simulink model "Target_Control_System"  (R2021b)
settings: Solver=FixedStepDiscrete  StartTime=0.0  StopTime=5  RelTol=1e-3
PreLoadFcn:
  | RTWConfigurationCB('preloadfcn', bdroot);
PostLoadFcn:
  | load('configuration/data_struct.mat');
  | load('configuration/fluxMaps_propMotor.mat');
  | load('configuration/parameterInit_PROP.mat');
  | load('configuration/parameterInit_PUMP.mat');
  | load('configuration/parameterInit_PITCH.mat');
  | load('configuration/parameterInit_TILT.mat');
  | %load('configuration/base_workspace_signal_definition.mat');
  | %load('resolvedatastores_to_baseworkspace_for_faster_simulation.mat');
model workspace (MAT data in the model file):
  SIMULATION_OPTIONS : Simulink.Parameter (value not decoded)
  TARGET_CODE_GEN : Simulink.Parameter (value not decoded)
  TCS_SAMPLE_FREQ_HZ : Simulink.Parameter (value not decoded)
symbols that are objects in the model workspace (value not decoded): TARGET_CODE_GEN, TCS_SAMPLE_FREQ_HZ
undefined symbols (not defined in the file): A_DQ_REF_LPF_INIT__PITCH, A_DQ_REF_LPF_INIT__PROP, A_DQ_REF_LPF_INIT__PUMP, A_DQ_REF_LPF_INIT__TILT, A_OBSERVER_CONFIDENCE_INIT__PITCH, A_OBSERVER_CONFIDENCE_INIT__PROP, A_OBSERVER_CONFIDENCE_INIT__PUMP, A_OBSERVER_CONFIDENCE_INIT__TILT, ACTUATOR_MAX_ANGLE_TRIP__PITCH, ACTUATOR_MIN_ANGLE_TRIP__PITCH, ACTUATOR_POS_SENSOR_INV_DIRECTION__PITCH, ACTUATOR_POS_SENSOR_INV_DIRECTION__TILT, ACTUATOR_POS_SENSOR_OFFSET__PITCH, ACTUATOR_POS_SENSOR_OFFSET__TILT, ADC_scaler1_baseaddr_TILT, ADC_SCALER_FLOAT_TO_FIXPOINT_EXPANSION, ANGLE_ELEC_FROM_SENSOR_OFFSET_INIT__PITCH, ANGLE_ELEC_FROM_SENSOR_OFFSET_INIT__PROP, ANGLE_ELEC_FROM_SENSOR_OFFSET_INIT__PUMP, ANGLE_ELEC_FROM_SENSOR_OFFSET_INIT__TILT, AUTO_CLEAR_FAULTS_ENABLED__PITCH, AUTO_CLEAR_FAULTS_ENABLED__PROP, AUTO_CLEAR_FAULTS_ENABLED__PUMP, AUTO_CLEAR_FAULTS_ENABLED__TILT, AUTO_CLEAR_FAULTS_WAIT_TICKS__PITCH, AUTO_CLEAR_FAULTS_WAIT_TICKS__PROP, AUTO_CLEAR_FAULTS_WAIT_TICKS__PUMP, AUTO_CLEAR_FAULTS_WAIT_TICKS__TILT, AUTO_I_ZERO_IDLE_TICKS__PITCH, AUTO_I_ZERO_IDLE_TICKS__PROP, AUTO_I_ZERO_IDLE_TICKS__PUMP, AUTO_I_ZERO_IDLE_TICKS__TILT, AUTO_I_ZERO_OFFSET_IDC_THRESHOLD__PITCH, AUTO_I_ZERO_OFFSET_IDC_THRESHOLD__PROP, AUTO_I_ZERO_OFFSET_IDC_THRESHOLD__PUMP, AUTO_I_ZERO_OFFSET_IDC_THRESHOLD__TILT, AUTO_I_ZERO_OFFSET_IPH_THRESHOLD__PITCH, AUTO_I_ZERO_OFFSET_IPH_THRESHOLD__PROP, AUTO_I_ZERO_OFFSET_IPH_THRESHOLD__PUMP, AUTO_I_ZERO_OFFSET_IPH_THRESHOLD__TILT, AUTO_SENSORLESS_SWITCHOVER_DISABLE_OMEGA, AUTO_SENSORLESS_SWITCHOVER_ENABLE_OMEGA, AUTO_SENSORLESS_SWITCHOVER_MIN_CONFIDENCE, AUXILIARY_PROTECTION_UNIT_BASEADDR__TILT, blanking_max_error_omega_INIT_PITCH, blanking_max_error_omega_INIT_TILT, blanking_max_error_position_INIT_PITCH, blanking_max_error_position_INIT_TILT, BRUTE_START_I_Q_REF_RAMP_SPEED__PITCH, BRUTE_START_I_Q_REF_RAMP_SPEED__PROP, BRUTE_START_I_Q_REF_RAMP_SPEED__PUMP, BRUTE_START_I_Q_REF_RAMP_SPEED__TILT, CONTROL_LOOP_DT_INIT__PITCH, CONTROL_LOOP_DT_INIT__PROP, CONTROL_LOOP_DT_INIT__PUMP, CONTROL_LOOP_DT_INIT__TILT, CORRECTION_FILTER_SCALE__PITCH, CORRECTION_FILTER_SCALE__PROP, CORRECTION_FILTER_SCALE__PUMP, CORRECTION_FILTER_SCALE__TILT ... (+458)
libraries: simulink x178, Reusables_Lib x24
(part 8 of 47)

== system Target_Control_System/Target_Control_System/InterruptFunction/tiltMotor_isrSchedule/Triggered Subsystem ==
  Trigger : TriggerPort  VariantControl=Variant
  Data Store Write6 : DataStoreWrite  Commented=on  DataStoreName=mdl_suiIsrSmallInvCounter_  IndexOptions=Index vector (dialog)  Indices=1  OutputSizes=1
  Function-Call Generator : simulink/Ports & Subsystems/Function-Call Generator  sample_time=-1  numberOfIterations=1  DisallowWideOutput=off
  constant : Constant  Commented=on  OutDataTypeStr=uint32  SampleTime=-1
  Output : Outport
  wires:
  constant/1 -> Data Store Write6/1
  Function-Call Generator/1 -> Output/1

== system Target_Control_System/Target_Control_System/InterruptFunction/tiltMotor_isrTask/abcToAlphaBeta ==
  abcToAlphaBeta : TriggerPort  TriggerType=function-call  VariantControl=Variant
  Alpha-Beta Calcs : Subsystem
  Calc Angle From Speed : Subsystem
  Constant1 : Constant  Value=TARGET_CODE_GEN  SampleTime=-1
  Data Store Read1 : DataStoreRead  DataStoreName=oTilt  DataStoreElements=oTilt.oIsr_.oIn_.oAdcData_.fIa_  IndexOptions=Index vector (dialog)  Indices=1  OutputSizes=1
  Data Store Read13 : DataStoreRead  DataStoreName=oTilt  DataStoreElements=oTilt.oIsr_.oParam_.iInverseDirection_  IndexOptions=Index vector (dialog)  Indices=1  OutputSizes=1
  Data Store Read14 : DataStoreRead  DataStoreName=oTilt  DataStoreElements=oTilt.oIsr_.oState_.fUaPostlpf_  IndexOptions=Index vector (dialog)  Indices=1  OutputSizes=1
  Data Store Read15 : DataStoreRead  DataStoreName=oTilt  DataStoreElements=oTilt.oIsr_.oState_.fUbPostlpf_  IndexOptions=Index vector (dialog)  Indices=1  OutputSizes=1
  Data Store Read16 : DataStoreRead  DataStoreName=oTilt  DataStoreElements=oTilt.oIsr_.oState_.fUcPostlpf_  IndexOptions=Index vector (dialog)  Indices=1  OutputSizes=1
  Data Store Read17 : DataStoreRead  DataStoreName=oTilt  DataStoreElements=oTilt.oIsr_.oState_.fOmegaEObserverRaw2_  IndexOptions=Index vector (dialog)  Indices=1  OutputSizes=1
  Data Store Read2 : DataStoreRead  DataStoreName=oTilt  DataStoreElements=oTilt.oIsr_.oIn_.oAdcData_.fIb_  IndexOptions=Index vector (dialog)  Indices=1  OutputSizes=1
  Data Store Read4 : DataStoreRead  DataStoreName=oTilt  DataStoreElements=oTilt.oIsr_.oIn_.oAdcData_.fIc_  IndexOptions=Index vector (dialog)  Indices=1  OutputSizes=1
  Data Store Read8 : DataStoreRead  DataStoreName=oTilt  DataStoreElements=oTilt.oIsr_.oIn_.fUphFilterDelayAngleRad_  IndexOptions=Index vector (dialog)  Indices=1  OutputSizes=1
  Data Store Write1 : DataStoreWrite  DataStoreName=oTilt  DataStoreElements=oTilt.oIsr_.oState_.fFluxMainAngleUltraRaw_  IndexOptions=Index vector (dialog)  Indices=1  OutputSizes=1
  Data Store Write2 : DataStoreWrite  DataStoreName=oTilt  DataStoreElements=oTilt.oIsr_.oState_.fIAlpha_  IndexOptions=Index vector (dialog)  Indices=1  OutputSizes=1
  Data Store Write3 : DataStoreWrite  DataStoreName=oTilt  DataStoreElements=oTilt.oIsr_.oState_.fIBeta_  IndexOptions=Index vector (dialog)  Indices=1  OutputSizes=1
  Data Store Write4 : DataStoreWrite  DataStoreName=oTilt  DataStoreElements=oTilt.oIsr_.oState_.fUAlpha_  IndexOptions=Index vector (dialog)  Indices=1  OutputSizes=1
  Data Store Write6 : DataStoreWrite  DataStoreName=oTilt  DataStoreElements=oTilt.oIsr_.oState_.fUBeta_  IndexOptions=Index vector (dialog)  Indices=1  OutputSizes=1
  ModelSource : Subsystem  Commented=on  Variant=on
  NOT1 : Logic  Operator=NOT  AllPortsSameDT=off  OutDataTypeStr=boolean
  vsincos()1 : Subsystem  TreatAsAtomicUnit=on
  wires:
  Alpha-Beta Calcs/4(fUBeta) -> Data Store Write6/1
  Data Store Read13/1 -> Alpha-Beta Calcs/1(iInverseDirection)
  Data Store Read16/1 -> Alpha-Beta Calcs/7(fUcPostlpf)
  Data Store Read1/1 -> Alpha-Beta Calcs/2(fIa)
  Alpha-Beta Calcs/3(fUAlpha) -> Data Store Write4/1
  Alpha-Beta Calcs/2(fIBeta) -> Data Store Write3/1
  Data Store Read15/1 -> Alpha-Beta Calcs/6(fUbPostlpf)
  Data Store Read17/1 -> Calc Angle From Speed/1(Omega)
  Data Store Read2/1 -> Alpha-Beta Calcs/3(fIb)
  Constant1/1 -> NOT1/1
  Data Store Read4/1 -> Alpha-Beta Calcs/4(fIc)
  Data Store Read8/1 -> vsincos()1/1(fUphFilterDelayAngleRad)
  Calc Angle From Speed/1(fFluxMainAngleRaw2) -> vsincos()1/2(fFluxMainAngleRaw2), Data Store Write1/1
  NOT1/1 -> vsincos()1/Enable
  Data Store Read14/1 -> Alpha-Beta Calcs/5(fUaPostlpf)
  Alpha-Beta Calcs/1(fIAlpha) -> Data Store Write2/1

== system Target_Control_System/Target_Control_System/InterruptFunction/tiltMotor_isrTask/currentController ==
  currentController : TriggerPort  TriggerType=function-call  VariantControl=Variant
  Data Store Read1 : DataStoreRead  DataStoreName=oTilt  DataStoreElements=oTilt.oIsr_.oIn_.uiCurrentControllerActive_  IndexOptions=Index vector (dialog)  Indices=1  OutputSizes=1
  Enabled Subsystem : Subsystem  TreatAsAtomicUnit=on
  wires:
  Data Store Read1/1 -> Enabled Subsystem/Enable

== system Target_Control_System/Target_Control_System/InterruptFunction/tiltMotor_isrTask/dqTransform ==
  dqTransform : TriggerPort  TriggerType=function-call  VariantControl=Variant
  DQ Transform : Subsystem
  Data Store Read4 : DataStoreRead  DataStoreName=oTilt  DataStoreElements=oTilt.oMot_.oParam_.fPolePairs_  IndexOptions=Index vector (dialog)  Indices=1  OutputSizes=1
  Data Store Read5 : DataStoreRead  DataStoreName=oTilt  DataStoreElements=oTilt.oIsr_.oState_.fFluxMainMagnitudeLpf_  IndexOptions=Index vector (dialog)  Indices=1  OutputSizes=1
  Data Store Read6 : DataStoreRead  DataStoreName=oTilt  DataStoreElements=oTilt.oIsr_.oState_.fIq_  IndexOptions=Index vector (dialog)  Indices=1  OutputSizes=1
  Data Store Read8 : DataStoreRead  DataStoreName=oTilt  DataStoreElements=oTilt.oIsr_.oState_.fIAlpha_  IndexOptions=Index vector (dialog)  Indices=1  OutputSizes=1
  Data Store Read9 : DataStoreRead  DataStoreName=oTilt  DataStoreElements=oTilt.oIsr_.oState_.fIBeta_  IndexOptions=Index vector (dialog)  Indices=1  OutputSizes=1
  Data Store Write1 : DataStoreWrite  DataStoreName=oTilt  DataStoreElements=oTilt.oIsr_.oOut_.fTEstimate_  IndexOptions=Index vector (dialog)  Indices=1  OutputSizes=1
  Data Store Write2 : DataStoreWrite  DataStoreName=oTilt  DataStoreElements=oTilt.oIsr_.oState_.fId_  IndexOptions=Index vector (dialog)  Indices=1  OutputSizes=1
  Data Store Write4 : DataStoreWrite  DataStoreName=oTilt  DataStoreElements=oTilt.oIsr_.oState_.fIq_  IndexOptions=Index vector (dialog)  Indices=1  OutputSizes=1
  Data Store Write5 : DataStoreWrite  DataStoreName=oTilt  DataStoreElements=oTilt.oIsr_.oOut_.fIPhaseMagnitude_  IndexOptions=Index vector (dialog)  Indices=1  OutputSizes=1
  Torque_Estimation_Pitch : Subsystem
  wires:
  DQ Transform/1(fId) -> Data Store Write2/1
  Data Store Read9/1 -> DQ Transform/2(fIBeta)
  DQ Transform/2(fIq) -> Data Store Write4/1
  Data Store Read4/1 -> Torque_Estimation_Pitch/1(fPolePairs)
  Torque_Estimation_Pitch/1(fTEstimate) -> Data Store Write1/1
  DQ Transform/3(fIPhaseMagnitude) -> Data Store Write5/1
  Data Store Read5/1 -> Torque_Estimation_Pitch/2(fFluxMainMagnitudeLpf)
  Data Store Read8/1 -> DQ Transform/1(fIAlpha)
  Data Store Read6/1 -> Torque_Estimation_Pitch/3(fIq)

== system Target_Control_System/Target_Control_System/InterruptFunction/tiltMotor_isrTask/fluxAngleCalculation ==
  fluxAngleCalculation : TriggerPort  TriggerType=function-call  VariantControl=Variant
  Advance Forced Angle : Subsystem
  Back Rotation : Subsystem
  Constant5 : Constant  Value=TARGET_CODE_GEN  SampleTime=-1
  Data Store Read10 : DataStoreRead  DataStoreName=oTilt  DataStoreElements=oTilt.oIsr_.oIn_.uiForcedAngle_  IndexOptions=Index vector (dialog)  Indices=1  OutputSizes=1
  Data Store Read2 : DataStoreRead  DataStoreName=oTilt  DataStoreElements=oTilt.oIsr_.oIn_.fOmegaERefRampOut_  IndexOptions=Index vector (dialog)  Indices=1  OutputSizes=1
  Data Store Read3 : DataStoreRead  DataStoreName=oTilt  DataStoreElements=oTilt.oIsr_.oParam_.iUseSensorAngle_  IndexOptions=Index vector (dialog)  Indices=1  OutputSizes=1
  Data Store Read4 : DataStoreRead  DataStoreName=oTilt  DataStoreElements=oTilt.oIsr_.oIn_.fFluxMasterAngleForced2closedSmoothingRampOut_  IndexOptions=Index vector (dialog)  Indices=1  OutputSizes=1
  Data Store Read5 : DataStoreRead  DataStoreName=oTilt  DataStoreElements=oTilt.oIsr_.oIn_.fOmegaElecFromPosSensor_  IndexOptions=Index vector (dialog)  Indices=1  OutputSizes=1
  Data Store Read6 : DataStoreRead  DataStoreName=oTilt  DataStoreElements=oTilt.oIsr_.oIn_.fFluxMasterAngleOffsetRampOut_  IndexOptions=Index vector (dialog)  Indices=1  OutputSizes=1
  Data Store Read7 : DataStoreRead  DataStoreName=oTilt  DataStoreElements=oTilt.oIsr_.oState_.fOmegaEObserverLpf2_  IndexOptions=Index vector (dialog)  Indices=1  OutputSizes=1
  Data Store Read8 : DataStoreRead  DataStoreName=oTilt  DataStoreElements=oTilt.oIsr_.oIn_.fAngleElecFromPosSensor_  IndexOptions=Index vector (dialog)  Indices=1  OutputSizes=1
  Data Store Read9 : DataStoreRead  DataStoreName=oTilt  DataStoreElements=oTilt.oIsr_.oState_.fFluxMainAngleRaw2_  IndexOptions=Index vector (dialog)  Indices=1  OutputSizes=1
  Data Store Write21 : DataStoreWrite  DataStoreName=mdl_tilt_fOmegaE  IndexOptions=Index vector (dialog)  Indices=1  OutputSizes=1
  Data Store Write3 : DataStoreWrite  DataStoreName=oTilt  DataStoreElements=oTilt.oIsr_.oState_.fFluxMasterAngleBkwd_  IndexOptions=Index vector (dialog)  Indices=1  OutputSizes=1
  Data Store Write4 : DataStoreWrite  DataStoreName=oTilt  DataStoreElements=oTilt.oIsr_.oState_.fFluxMasterAngle_  IndexOptions=Index vector (dialog)  Indices=1  OutputSizes=1
  Equal4 : RelationalOperator  Operator===  OutDataTypeStr=boolean  RndMeth=Simplest
  ModelSource : Subsystem  Variant=on
  NOT2 : Logic  Operator=NOT  AllPortsSameDT=off  OutDataTypeStr=boolean
  Not forced Angle : Subsystem
  One3 : Constant  OutDataTypeStr=uint32  SampleTime=-1
  Switch1 : Switch  Criteria=u2 > Threshold  Threshold=0.5
  Switch2 : Switch  Criteria=u2 > Threshold  Threshold=0.5
  vsincos() : Subsystem  TreatAsAtomicUnit=on
  wires:
  Constant5/1 -> NOT2/1
  Advance Forced Angle/1(Output) -> Switch2/1
  Data Store Read2/1 -> Advance Forced Angle/1(Input), Switch1/1
  Equal4/1 -> Switch1/2, Switch2/2
  Data Store Read3/1 -> Not forced Angle/1(iUseSensorAngle)
  Switch2/1 -> Data Store Write4/1, vsincos()/2(fFluxMasterAngle), Back Rotation/2(fFluxMasterAngle)
  Data Store Read6/1 -> Back Rotation/1(fFluxMasterAngleOffsetRampOut)
  One3/1 -> Equal4/2
  Data Store Read4/1 -> Not forced Angle/6(fFluxMasterAngleForced2closedSmoothingRampOut)
  Data Store Read5/1 -> Not forced Angle/4(fOmegaElecFromPosSensor)
  Data Store Read7/1 -> Not forced Angle/5(fOmegaEObserverLpf2)
  Data Store Read9/1 -> Not forced Angle/3(fFluxMainAngleRaw2)
  Data Store Read8/1 -> Not forced Angle/2(fAngleElecFromPosSensor)
  Data Store Read10/1 -> Equal4/1
  Not forced Angle/1(fFluxMasterAngle) -> Switch2/3
  Back Rotation/1(fFluxMasterAngleBkwd) -> Data Store Write3/1, vsincos()/1(fFluxMasterAngleBkwd)
  Switch1/1 -> Data Store Write21/1
  NOT2/1 -> vsincos()/Enable
  Not forced Angle/2(fOmegaE) -> Switch1/3

== system Target_Control_System/Target_Control_System/InterruptFunction/tiltMotor_isrTask/fluxObserver ==
  fluxObserver : TriggerPort  TriggerType=function-call  VariantControl=Variant
  Calculate Coil Flux + Bleeder : Subsystem
  Calculate Main Flux + LPF : Subsystem
  Data Store Read : DataStoreRead  DataStoreName=oTilt  DataStoreElements=oTilt.oIsr_.oParam_.fRsPhase_  IndexOptions=Index vector (dialog)  Indices=1  OutputSizes=1
  Data Store Read1 : DataStoreRead  DataStoreName=oTilt  DataStoreElements=oTilt.oIsr_.oIn_.fUphFilterAmplitudeRatio_  IndexOptions=Index vector (dialog)  Indices=1  OutputSizes=1
  Data Store Read10 : DataStoreRead  DataStoreName=oTilt  DataStoreElements=oTilt.oIsr_.oParam_.fLsPhase_  IndexOptions=Index vector (dialog)  Indices=1  OutputSizes=1
  Data Store Read11 : DataStoreRead  DataStoreName=oTilt  DataStoreElements=oTilt.oMot_.oParam_.fObserverLoopFilterBandwidthHz_  IndexOptions=Index vector (dialog)  Indices=1  OutputSizes=1
  Data Store Read12 : DataStoreRead  DataStoreName=oTilt  DataStoreElements=oTilt.oIsr_.oParam_.oPiDataPll2_.fState_  IndexOptions=Index vector (dialog)  Indices=1  OutputSizes=1
  Data Store Read13 : DataStoreRead  DataStoreName=oTilt  DataStoreElements=oTilt.oIsr_.oParam_.oPiDataPll2_.oParameter_.fKp_  IndexOptions=Index vector (dialog)  Indices=1  OutputSizes=1
  Data Store Read14 : DataStoreRead  DataStoreName=oTilt  DataStoreElements=oTilt.oIsr_.oParam_.oPiDataPll2_.oParameter_.fKi_  IndexOptions=Index vector (dialog)  Indices=1  OutputSizes=1
  Data Store Read15 : DataStoreRead  DataStoreName=oTilt  DataStoreElements=oTilt.oIsr_.oParam_.oPiDataPll2_.oParameter_.fLoopDt_  IndexOptions=Index vector (dialog)  Indices=1  OutputSizes=1
  Data Store Read16 : DataStoreRead  DataStoreName=oTilt  DataStoreElements=oTilt.oIsr_.oParam_.oPiDataPll2_.oParameter_.fIntMax_  IndexOptions=Index vector (dialog)  Indices=1  OutputSizes=1
  Data Store Read17 : DataStoreRead  DataStoreName=oTilt  DataStoreElements=oTilt.oIsr_.oParam_.oPiDataPll2_.oParameter_.fOutMax_  IndexOptions=Index vector (dialog)  Indices=1  OutputSizes=1
  Data Store Read18 : DataStoreRead  DataStoreName=oTilt  DataStoreElements=oTilt.oIsr_.oParam_.oPiDataPll2_.oParameter_.fIntMin_  IndexOptions=Index vector (dialog)  Indices=1  OutputSizes=1
  Data Store Read19 : DataStoreRead  DataStoreName=oTilt  DataStoreElements=oTilt.oIsr_.oParam_.oPiDataPll2_.oParameter_.fOutMin_  IndexOptions=Index vector (dialog)  Indices=1  OutputSizes=1
  Data Store Read2 : DataStoreRead  DataStoreName=mdl_tilt_fFluxMainAngleRaw2_sin_  IndexOptions=Index vector (dialog)  Indices=1  OutputSizes=1
  Data Store Read27 : DataStoreRead  DataStoreName=mdl_tilt_fUphFilterDelayAngleRad_sin_  IndexOptions=Index vector (dialog)  Indices=1  OutputSizes=1
  Data Store Read28 : DataStoreRead  DataStoreName=mdl_tilt_fUphFilterDelayAngleRad_cos_  IndexOptions=Index vector (dialog)  Indices=1  OutputSizes=1
  Data Store Read3 : DataStoreRead  DataStoreName=oTilt  DataStoreElements=oTilt.oIsr_.oParam_.uiUphFilterCorrectionEnabled_  IndexOptions=Index vector (dialog)  Indices=1  OutputSizes=1
  Data Store Read34 : DataStoreRead  DataStoreName=mdl_tilt_fFluxMainAngleRaw2_cos_  IndexOptions=Index vector (dialog)  Indices=1  OutputSizes=1
  Data Store Read4 : DataStoreRead  DataStoreName=oTilt  DataStoreElements=oTilt.oIsr_.oState_.fUAlpha_  IndexOptions=Index vector (dialog)  Indices=1  OutputSizes=1
  Data Store Read5 : DataStoreRead  DataStoreName=oTilt  DataStoreElements=oTilt.oIsr_.oState_.fUBeta_  IndexOptions=Index vector (dialog)  Indices=1  OutputSizes=1
  Data Store Read6 : DataStoreRead  DataStoreName=oTilt  DataStoreElements=oTilt.oIsr_.oState_.fIAlpha_  IndexOptions=Index vector (dialog)  Indices=1  OutputSizes=1
  Data Store Read7 : DataStoreRead  DataStoreName=oTilt  DataStoreElements=oTilt.oIsr_.oState_.fIBeta_  IndexOptions=Index vector (dialog)  Indices=1  OutputSizes=1
  Data Store Read8 : DataStoreRead  DataStoreName=oTilt  DataStoreElements=oTilt.oIsr_.oParam_.fControlLoopDt_  IndexOptions=Index vector (dialog)  Indices=1  OutputSizes=1
  Data Store Read9 : DataStoreRead  DataStoreName=oTilt  DataStoreElements=oTilt.oIsr_.oParam_.fKFluxBleeder_  IndexOptions=Index vector (dialog)  Indices=1  OutputSizes=1
  Data Store Write1 : DataStoreWrite  DataStoreName=oTilt  DataStoreElements=oTilt.oIsr_.oState_.fFluxCoilAlpha_  IndexOptions=Index vector (dialog)  Indices=1  OutputSizes=1
  Data Store Write10 : DataStoreWrite  DataStoreName=oTilt  DataStoreElements=oTilt.oIsr_.oState_.fAtan2loopfilter2Out_  IndexOptions=Index vector (dialog)  Indices=1  OutputSizes=1
  Data Store Write11 : DataStoreWrite  DataStoreName=oTilt  DataStoreElements=oTilt.oIsr_.oParam_.oPiDataPll2_.fState_  IndexOptions=Index vector (dialog)  Indices=1  OutputSizes=1
  Data Store Write12 : DataStoreWrite  DataStoreName=oTilt  DataStoreElements=oTilt.oIsr_.oState_.fOmegaEObserverRaw2_  IndexOptions=Index vector (dialog)  Indices=1  OutputSizes=1
  Data Store Write13 : DataStoreWrite  DataStoreName=oTilt  DataStoreElements=oTilt.oIsr_.oState_.fOmegaEObserverLpf2_  IndexOptions=Index vector (dialog)  Indices=1  OutputSizes=1
  Data Store Write14 : DataStoreWrite  DataStoreName=oTilt  DataStoreElements=oTilt.oIsr_.oState_.fFluxMainMagnitudeLpf_  IndexOptions=Index vector (dialog)  Indices=1  OutputSizes=1
  Data Store Write15 : DataStoreWrite  DataStoreName=oTilt  DataStoreElements=oTilt.oIsr_.oState_.fFluxMainMagnitude_  IndexOptions=Index vector (dialog)  Indices=1  OutputSizes=1
  Data Store Write2 : DataStoreWrite  DataStoreName=oTilt  DataStoreElements=oTilt.oIsr_.oState_.fUBeta_  IndexOptions=Index vector (dialog)  Indices=1  OutputSizes=1
  Data Store Write28 : DataStoreWrite  DataStoreName=oTilt  DataStoreElements=oTilt.oIsr_.oState_.fIAlphaLpf4hpf_  IndexOptions=Index vector (dialog)  Indices=1  OutputSizes=1
  Data Store Write29 : DataStoreWrite  DataStoreName=oTilt  DataStoreElements=oTilt.oIsr_.oState_.fIBetaLpf4hpf_  IndexOptions=Index vector (dialog)  Indices=1  OutputSizes=1
  Data Store Write3 : DataStoreWrite  DataStoreName=oTilt  DataStoreElements=oTilt.oIsr_.oState_.fUAlphaLpf4hpf_  IndexOptions=Index vector (dialog)  Indices=1  OutputSizes=1
  Data Store Write4 : DataStoreWrite  DataStoreName=oTilt  DataStoreElements=oTilt.oIsr_.oState_.fUBetaLpf4hpf_  IndexOptions=Index vector (dialog)  Indices=1  OutputSizes=1
  Data Store Write5 : DataStoreWrite  DataStoreName=oTilt  DataStoreElements=oTilt.oIsr_.oState_.fUAlpha_  IndexOptions=Index vector (dialog)  Indices=1  OutputSizes=1
  Data Store Write6 : DataStoreWrite  DataStoreName=oTilt  DataStoreElements=oTilt.oIsr_.oState_.fFluxCoilBeta_  IndexOptions=Index vector (dialog)  Indices=1  OutputSizes=1
  Data Store Write7 : DataStoreWrite  DataStoreName=oTilt  DataStoreElements=oTilt.oIsr_.oState_.fFluxMainAlpha_  IndexOptions=Index vector (dialog)  Indices=1  OutputSizes=1
  Data Store Write8 : DataStoreWrite  DataStoreName=oTilt  DataStoreElements=oTilt.oIsr_.oState_.fFluxMainBeta_  IndexOptions=Index vector (dialog)  Indices=1  OutputSizes=1
  Data Store Write9 : DataStoreWrite  DataStoreName=oTilt  DataStoreElements=oTilt.oIsr_.oState_.fFluxMainAngleUltraRaw_  IndexOptions=Index vector (dialog)  Indices=1  OutputSizes=1
  Fast PLL : Subsystem
  HPF Currents : Subsystem
  HPF Voltages : Subsystem
  Mux : Mux  Inputs=7
  Subtract Resistive Voltage Drop : Subsystem
  Ultra Raw Angle : Subsystem
  Voltage Vector Rotation : Subsystem
  wires:
  Data Store Read13/1 -> Mux/1
  Data Store Read5/1 -> Voltage Vector Rotation/6(fUBeta)
  Calculate Main Flux + LPF/2(fFluxMainBeta) -> Fast PLL/4(fFluxMainBeta), Ultra Raw Angle/2(fFluxMainBeta), Data Store Write8/1
  Data Store Read11/1 -> Fast PLL/5(fObserverLoopFilterBandwidthHz)
  Voltage Vector Rotation/2(fUBeta_out) -> Subtract Resistive Voltage Drop/5(fUBeta)
  Data Store Read34/1 -> Fast PLL/2(fluxAngle_cos)
  Data Store Read27/1 -> Voltage Vector Rotation/1(UphFilterDelayAngleRad_sin)
  Fast PLL/1(fAtan2loopfilter2Out) -> Data Store Write10/1
  HPF Currents/2(fIBetaLpf4hpf) -> Data Store Write29/1
  Calculate Coil Flux + Bleeder/1(fFluxCoilAlpha) -> Calculate Main Flux + LPF/4(fFluxCoilAlpha), Data Store Write1/1
  Data Store Read14/1 -> Mux/2
  Data Store Read3/1 -> Voltage Vector Rotation/4(uiUphFilterCorrectionEnabled)
  Data Store Read10/1 -> Calculate Main Flux + LPF/3(fLsPhase)
  Data Store Read7/1 -> HPF Currents/2(fIBeta)
  Data Store Read1/1 -> Voltage Vector Rotation/3(fUphFilterAmplitudeRatio)
  Data Store Read2/1 -> Fast PLL/1(fluxAngle_sin)
  Data Store Read/1 -> Subtract Resistive Voltage Drop/3(fRsPhase)
  HPF Currents/4(fIBetaLocal) -> Calculate Main Flux + LPF/2(fIBetaLocal), Subtract Resistive Voltage Drop/2(fIBetaLocal)  "fIBetaLocal"
  Data Store Read18/1 -> Mux/6
  Calculate Coil Flux + Bleeder/2(fFluxCoilBeta) -> Calculate Main Flux + LPF/5(fFluxCoilBeta), Data Store Write6/1
  Calculate Main Flux + LPF/3(fFluxMainMagnitude) -> Data Store Write15/1
  Subtract Resistive Voltage Drop/2(fUBeta_out) -> HPF Voltages/2(fUBeta)
  Fast PLL/4(fOmegaEObserverLpf2) -> Data Store Write13/1
  Data Store Read4/1 -> Voltage Vector Rotation/5(fUAlpha)
  Data Store Read9/1 -> Calculate Coil Flux + Bleeder/2(fKFluxBleeder)
  Fast PLL/2(oPiDataPll2_.fState*) -> Data Store Write11/1
  Data Store Read28/1 -> Voltage Vector Rotation/2(UphFilterDelayAngleRad_cos)
  Data Store Read16/1 -> Mux/4
  Data Store Read8/1 -> Calculate Coil Flux + Bleeder/1(fControlLoopDt)
  Subtract Resistive Voltage Drop/1(fUAlpha_out) -> HPF Voltages/1(fUAlpha)
  Fast PLL/3(fOmegaEObserverRaw2) -> Data Store Write12/1
  HPF Currents/3(fIAlphaLocal) -> Calculate Main Flux + LPF/1(fIAlphaLocal), Subtract Resistive Voltage Drop/1(fIAlphaLocal)  "fIAlphaLocal"
  Data Store Read19/1 -> Mux/7
  HPF Voltages/1(fUAlphaLpf4hpf) -> Data Store Write3/1
  Data Store Read6/1 -> HPF Currents/1(fIAlpha)
  Mux/1 -> Fast PLL/7(oPiDataPll2_.oParameter)
  HPF Voltages/4(fUBeta_out) -> Calculate Coil Flux + Bleeder/4(fUBeta), Data Store Write2/1
  Calculate Main Flux + LPF/4(fFluxMainMagnitudeLpf) -> Data Store Write14/1
  Calculate Main Flux + LPF/1(fFluxMainAlpha) -> Data Store Write7/1, Fast PLL/3(fFluxMainAlpha), Ultra Raw Angle/1(fFluxMainAlpha)
  HPF Currents/1(fIAlphaLpf4hpf) -> Data Store Write28/1
  HPF Voltages/2(fUBetaLpf4hpf) -> Data Store Write4/1
  Data Store Read15/1 -> Mux/3
  Voltage Vector Rotation/1(fUAlpha_out) -> Subtract Resistive Voltage Drop/4(fUAlpha)
  Ultra Raw Angle/1(fFluxMainAngleUltraRaw) -> Data Store Write9/1
  Data Store Read17/1 -> Mux/5
  Data Store Read12/1 -> Fast PLL/6(oPiDataPll2_.fState)
  HPF Voltages/3(fUAlpha_out) -> Data Store Write5/1, Calculate Coil Flux + Bleeder/3(fUAlpha)

== system Target_Control_System/Target_Control_System/InterruptFunction/tiltMotor_isrTask/isrStateMachine ==
  isrStateMachine : TriggerPort  TriggerType=function-call  VariantControl=Variant
  ISR State Machine : Stateflow chart  TreatAsAtomicUnit=on

== system Target_Control_System/Target_Control_System/InterruptFunction/tiltMotor_isrTask/pwmGeneration ==
  pwmGeneration : TriggerPort  TriggerType=function-call  VariantControl=Variant
  Data Store Read1 : DataStoreRead  DataStoreName=oTilt  DataStoreElements=oTilt.oIsr_.oIn_.uiCurrentControllerActive_  IndexOptions=Index vector (dialog)  Indices=1  OutputSizes=1
  Subsystem : Subsystem
  wires:
  Data Store Read1/1 -> Subsystem/Enable

== system Target_Control_System/Target_Control_System/InterruptFunction/tiltMotor_isrTask/resetFlags ==
  resetFlags : TriggerPort  TriggerType=function-call  VariantControl=Variant
  Constant : Constant  Value=0  OutDataTypeStr=int32  SampleTime=-1
  Data Store Write1 : DataStoreWrite  DataStoreName=oTilt  DataStoreElements=oTilt.oIsr_.oState_.iPwmUpdated_  IndexOptions=Index vector (dialog)  Indices=1  OutputSizes=1
  Data Store Write2 : DataStoreWrite  DataStoreName=oTilt  DataStoreElements=oTilt.oIsr_.oOut_.iIBiasUpdated_  IndexOptions=Index vector (dialog)  Indices=1  OutputSizes=1
  Data Store Write3 : DataStoreWrite  DataStoreName=oTilt  DataStoreElements=oTilt.oIsr_.oOut_.iUBiasUpdated_  IndexOptions=Index vector (dialog)  Indices=1  OutputSizes=1
  wires:
  Constant/1 -> Data Store Write1/1, Data Store Write2/1, Data Store Write3/1

== system Target_Control_System/Target_Control_System/InterruptFunction/tiltMotor_isrTask/softCurrentLimiting ==
  softCurrentLimiting : TriggerPort  TriggerType=function-call  VariantControl=Variant

== system Target_Control_System/Target_Control_System/InterruptFunction/tiltMotor_setPwm/ModelSourceFPGATilt ==
  note: 1) Add Subsystem or Model blocks as valid variant choices.
      | 2) You cannot connect blocks at this level. At simulation, connectivity is automatically
      | determined, based on the active variant and port name matching.
  DoNotIncludeCustomCode : Subsystem  TreatAsAtomicUnit=on  VariantControl=TARGET_CODE_GEN == 0
  IncludeCustomCode : Subsystem  TreatAsAtomicUnit=on  VariantControl=(default)

== system Target_Control_System/Target_Control_System/InterruptFunction/tiltMotor_setPwm/Subsystem ==
  note: // signal to the pwm block that we handled the interrupt
  Enable : EnablePort
  Constant10 : Constant  OutDataTypeStr=int32  SampleTime=-1
  Data Store Read2 : DataStoreRead  DataStoreName=oTilt  DataStoreElements=oTilt.oIsr_.oParam_.fPwmPeriodTicksFloat_  IndexOptions=Index vector (dialog)  Indices=1  OutputSizes=1
  Data Store Write : DataStoreWrite  DataStoreName=oTilt  DataStoreElements=oTilt.oIsr_.oOut_.uiPwmDutyTicksA_  IndexOptions=Index vector (dialog)  Indices=1  OutputSizes=1
  Data Type Conversion : DataTypeConversion  OutDataTypeStr=uint32
  Shift Arithmetic1 : ArithShift  BitShiftNumberSource=Input port  BitShiftNumber=8  BitShiftDirection=Right
      settings: InputPortMap=u0,p1
  wires:
  Shift Arithmetic1/1 -> Data Type Conversion/1
  Data Type Conversion/1 -> Data Store Write/1
  Data Store Read2/1 -> Shift Arithmetic1/1
  Constant10/1 -> Shift Arithmetic1/2

== system Target_Control_System/Target_Control_System/MainLoop/pitchMotor_mainLoop/Decimation gate for 10 Hz Pitch ==
  Function-Call Generator : simulink/Ports & Subsystems/Function-Call Generator  sample_time=-1  numberOfIterations=1  DisallowWideOutput=off
  Function-Call Subsystem : Subsystem  TreatAsAtomicUnit=on
  Idle-Loop State Machine Pitch : Stateflow chart  TreatAsAtomicUnit=on
  wires:
  Function-Call Generator/1 -> Function-Call Subsystem/Trigger

== system Target_Control_System/Target_Control_System/MainLoop/pitchMotor_mainLoop/Decimation gate for 200 Hz Pitch ==
  Function-Call Generator : simulink/Ports & Subsystems/Function-Call Generator  sample_time=-1  numberOfIterations=1  DisallowWideOutput=off
  Function-Call Subsystem : Subsystem  TreatAsAtomicUnit=on
  wires:
  Function-Call Generator/1 -> Function-Call Subsystem/Trigger

== system Target_Control_System/Target_Control_System/MainLoop/pitchMotor_mainLoop/Decimation gate for 5000 Hz Pitch ==
  Function-Call Generator : simulink/Ports & Subsystems/Function-Call Generator  sample_time=-1  numberOfIterations=1  DisallowWideOutput=off
  motorTaskProcessExternalSetpoints(&oPitch) : Subsystem  TreatAsAtomicUnit=on
  wires:
  Function-Call Generator/1 -> motorTaskProcessExternalSetpoints(&oPitch)/Trigger

== system Target_Control_System/Target_Control_System/MainLoop/pitchMotor_mainLoop/mainTask_pitch ==
  Constant4 : Constant  Value=TARGET_CODE_GEN  SampleTime=-1
  Function-Call Split1 : FunctionCallSplit  NumOutputPorts=2
  Function-Call Split10 : FunctionCallSplit  NumOutputPorts=2
  NOT : Logic  Operator=NOT  IconShape=distinctive  AllPortsSameDT=off  OutDataTypeStr=boolean
  PWM for Simulation : Subsystem  TreatAsAtomicUnit=on
  Variant Subsystem : Subsystem  Variant=on
  motorTaskMainFastStep() : Subsystem
  motorTaskManagePwmRequestFlags() : Subsystem
  resetFlag_uiDataFromIsrToMainUpdated : Subsystem
  Out1 : Outport
  wires:
  PWM for Simulation/1(Out1) -> Out1/1  "pitchMotor_PWMticks"
  NOT/1 -> PWM for Simulation/Enable
  Constant4/1 -> NOT/1
  Function-Call Split10/1 -> motorTaskMainFastStep()/Trigger
  Variant Subsystem/1(Output) -> Function-Call Split10/1
  Function-Call Split1/2 -> resetFlag_uiDataFromIsrToMainUpdated/Trigger
  Function-Call Split1/1 -> motorTaskManagePwmRequestFlags()/Trigger
  Function-Call Split10/2 -> Function-Call Split1/1

== system Target_Control_System/Target_Control_System/MainLoop/propMotor_mainLoop/Decimation gate A for 200 Hz Prop ==
  Cross-tripping VP/Tilt to Prop : Subsystem  Commented=on
  Current offset nulling : Subsystem  TreatAsAtomicUnit=on
  Function-Call Generator : simulink/Ports & Subsystems/Function-Call Generator  sample_time=-1  numberOfIterations=1  DisallowWideOutput=off
  Function-Call Split : FunctionCallSplit  NumOutputPorts=2  OutputPortLayout=default
  Subsystem : Subsystem
  wires:
  Function-Call Split/1 -> Subsystem/Trigger
  Function-Call Generator/1 -> Function-Call Split/1
  Function-Call Split/2 -> Current offset nulling/Trigger

== system Target_Control_System/Target_Control_System/MainLoop/propMotor_mainLoop/Decimation gate for 5000 Hz Prop ==
  Function-Call Generator : simulink/Ports & Subsystems/Function-Call Generator  sample_time=-1  numberOfIterations=1  DisallowWideOutput=off
  motorTaskProcessExternalSetpoints(&oProp) : Subsystem  TreatAsAtomicUnit=on
  wires:
  Function-Call Generator/1 -> motorTaskProcessExternalSetpoints(&oProp)/Trigger

== system Target_Control_System/Target_Control_System/MainLoop/propMotor_mainLoop/motorStateMachineLogic(&oProp) ==
  Idle-Loop State Machine Prop : Stateflow chart  TreatAsAtomicUnit=on

== system Target_Control_System/Target_Control_System/MainLoop/propMotor_mainLoop/motorTaskMainFastStep(&oProp) ==
  Compare To Constant : simulink/Logic and Bit Operations/Compare To Constant  relop=<  const=20  OutDataTypeStr=boolean
  Compare To Constant1 : simulink/Logic and Bit Operations/Compare To Constant  relop=<  const=20  OutDataTypeStr=boolean
  Constant : Constant  Value=20  OutDataTypeStr=single  SampleTime=-1
  Constant2 : Constant  Value=20  OutDataTypeStr=single  SampleTime=-1
  Constant7 : Constant  Value=TARGET_CODE_GEN  SampleTime=-1
  Control Loops - Prop : Subsystem
  Correction Constants for Observer and Control - Prop : Subsystem
  Data Store Read25 : DataStoreRead  DataStoreName=oProp  DataStoreElements=oProp.oMot_.oIn_.oAdcData_.fUdc_  IndexOptions=Index vector (dialog)  Indices=1  OutputSizes=1
  Data Store Read32 : DataStoreRead  DataStoreName=oPump  DataStoreElements=oPump.oMot_.oIn_.oAdcData_.fUdc_  IndexOptions=Index vector (dialog)  Indices=1  OutputSizes=1
  Data Store Write12 : DataStoreWrite  DataStoreName=oPitch  DataStoreElements=oPitch.oMot_.oOut_.fOneOverUdc_  IndexOptions=Index vector (dialog)  Indices=1  OutputSizes=1
  Data Store Write13 : DataStoreWrite  DataStoreName=oTilt  DataStoreElements=oTilt.oMot_.oOut_.fOneOverUdc_  IndexOptions=Index vector (dialog)  Indices=1  OutputSizes=1
  Data Store Write5 : DataStoreWrite  DataStoreName=oPump  DataStoreElements=oPump.oMot_.oOut_.fOneOverUdc_  IndexOptions=Index vector (dialog)  Indices=1  OutputSizes=1
  Data Store Write6 : DataStoreWrite  DataStoreName=oProp  DataStoreElements=oProp.oMot_.oOut_.fOneOverUdc_  IndexOptions=Index vector (dialog)  Indices=1  OutputSizes=1
  Function-Call Generator : simulink/Ports & Subsystems/Function-Call Generator  sample_time=-1  numberOfIterations=1  DisallowWideOutput=off
  Function-Call Split{1..4,10} (5 alike) : FunctionCallSplit  NumOutputPorts=2
  IsNaN : RelationalOperator  Operator=isNaN  OutDataTypeStr=boolean  RndMeth=Simplest
  IsNaN1 : RelationalOperator  Operator=isNaN  OutDataTypeStr=boolean  RndMeth=Simplest
  Lowpass Filtered Quantities for External World - Prop : Subsystem
  NOT : Logic  Operator=NOT  IconShape=distinctive  AllPortsSameDT=off  OutDataTypeStr=boolean
  OR : Logic  Operator=OR  AllPortsSameDT=off  OutDataTypeStr=boolean
  OR1 : Logic  Operator=OR  AllPortsSameDT=off  OutDataTypeStr=boolean
  Observer Confidence - Prop : Subsystem
  One_Over : Fcn  Expr=1/u
  One_Over2 : Fcn  Expr=1/u
  PWM for Simulation : Subsystem  TreatAsAtomicUnit=on
  Switch2 : Switch  Criteria=u2 > Threshold  OutDataTypeStr=single
  Switch4 : Switch  Criteria=u2 > Threshold  OutDataTypeStr=single
  enableDrive(&oProp) : Stateflow chart  TreatAsAtomicUnit=on
  initiateOffsetNulling(&oProp) : Stateflow chart  TreatAsAtomicUnit=on
  motorTaskManagePwmRequestFlags() : Subsystem
  resetFlag_uiDataFromIsrToMainUpdated : Subsystem
  Motor : Outport
  wires:
  Function-Call Split3/2 -> Function-Call Split4/1
  Function-Call Split3/1 -> Correction Constants for Observer and Control - Prop/Trigger
  Function-Call Split2/2 -> Function-Call Split3/1
  Function-Call Split4/1 -> motorTaskManagePwmRequestFlags()/Trigger
  Function-Call Split4/2 -> resetFlag_uiDataFromIsrToMainUpdated/Trigger
  Constant/1 -> Switch2/1
  Compare To Constant1/1 -> OR1/2
  Data Store Read25/1 -> Switch2/3, Compare To Constant/1, IsNaN/1
  Constant2/1 -> Switch4/1
  IsNaN/1 -> OR/1
  Switch2/1 -> One_Over/1  "Ua"
  Data Store Read32/1 -> Switch4/3, Compare To Constant1/1, IsNaN1/1
  One_Over/1 -> Data Store Write6/1
  OR1/1 -> Switch4/2
  One_Over2/1 -> Data Store Write5/1, Data Store Write12/1, Data Store Write13/1
  OR/1 -> Switch2/2
  Switch4/1 -> One_Over2/1  "Ua"
  IsNaN1/1 -> OR1/1
  Compare To Constant/1 -> OR/2
  Function-Call Generator/1 -> Function-Call Split10/1
  Function-Call Split2/1 -> Control Loops - Prop/Trigger
  Function-Call Split1/2 -> Function-Call Split2/1
  Function-Call Split10/1 -> Observer Confidence - Prop/Trigger
  Function-Call Split10/2 -> Function-Call Split1/1
  Function-Call Split1/1 -> Lowpass Filtered Quantities for External World - Prop/Trigger
  PWM for Simulation/1(Motor) -> Motor/1  "propMotor_PWMticks"
  Constant7/1 -> NOT/1
  NOT/1 -> PWM for Simulation/Enable

== system Target_Control_System/Target_Control_System/MainLoop/pumpMotor_mainLoop/Decimation gate A for 200 Hz Pump ==
  Current offset nulling : Subsystem  TreatAsAtomicUnit=on
  Function-Call Generator : simulink/Ports & Subsystems/Function-Call Generator  sample_time=-1  numberOfIterations=1  DisallowWideOutput=off
  Function-Call Split : FunctionCallSplit  NumOutputPorts=2  OutputPortLayout=default
  Subsystem : Subsystem
  wires:
  Function-Call Split/1 -> Subsystem/Trigger
  Function-Call Generator/1 -> Function-Call Split/1
  Function-Call Split/2 -> Current offset nulling/Trigger

== system Target_Control_System/Target_Control_System/MainLoop/pumpMotor_mainLoop/Decimation gate for 5000 Hz Pump ==
  Function-Call Generator : simulink/Ports & Subsystems/Function-Call Generator  sample_time=-1  numberOfIterations=1  DisallowWideOutput=off
  motorTaskProcessExternalSetpoints(&oPump) : Subsystem  TreatAsAtomicUnit=on
  wires:
  Function-Call Generator/1 -> motorTaskProcessExternalSetpoints(&oPump)/Trigger

== system Target_Control_System/Target_Control_System/MainLoop/pumpMotor_mainLoop/motorStateMachineLogic(&oPump) ==
  Idle-Loop State Machine Pump : Stateflow chart  TreatAsAtomicUnit=on

== system Target_Control_System/Target_Control_System/MainLoop/pumpMotor_mainLoop/motorTaskMainFastStep(&oPump) ==
  Constant2 : Constant  Value=TARGET_CODE_GEN  SampleTime=-1
  Control Loops - Pump : Subsystem
  Correction Constants for Observer and Control - Pump : Subsystem
  Function-Call Split{1..4,10} (5 alike) : FunctionCallSplit  NumOutputPorts=2
  Lowpass Filtered Quantities for External World - Pump : Subsystem
  NOT : Logic  Operator=NOT  IconShape=distinctive  AllPortsSameDT=off  OutDataTypeStr=boolean
  Observer Confidence - Pump : Subsystem
  PWM for Simulation : Subsystem  TreatAsAtomicUnit=on
  Variant Subsystem : Subsystem  Variant=on
  enableDrive(&oPump) : Stateflow chart  TreatAsAtomicUnit=on
  initiateOffsetNulling(&oPump) : Stateflow chart  TreatAsAtomicUnit=on
  motorTaskManagePwmRequestFlags() : Subsystem
  resetFlag_uiDataFromIsrToMainUpdated : Subsystem
  Motor : Outport
  wires:
  Function-Call Split4/2 -> resetFlag_uiDataFromIsrToMainUpdated/Trigger
  Function-Call Split4/1 -> motorTaskManagePwmRequestFlags()/Trigger
  Function-Call Split3/2 -> Function-Call Split4/1
  Function-Call Split3/1 -> Correction Constants for Observer and Control - Pump/Trigger
  Function-Call Split2/2 -> Function-Call Split3/1
  Function-Call Split1/2 -> Function-Call Split2/1
  Function-Call Split2/1 -> Control Loops - Pump/Trigger
  Function-Call Split1/1 -> Lowpass Filtered Quantities for External World - Pump/Trigger
  Function-Call Split10/1 -> Observer Confidence - Pump/Trigger
  Function-Call Split10/2 -> Function-Call Split1/1
  Variant Subsystem/1(Output) -> Function-Call Split10/1
  PWM for Simulation/1(Motor) -> Motor/1  "pumpMotor_PWMticks"
  NOT/1 -> PWM for Simulation/Enable
  Constant2/1 -> NOT/1

== system Target_Control_System/Target_Control_System/MainLoop/tiltMotor_mainLoop/Decimation gate for 10 Hz Tilt ==
  Function-Call Generator : simulink/Ports & Subsystems/Function-Call Generator  sample_time=-1  numberOfIterations=1  DisallowWideOutput=off
  Function-Call Subsystem : Subsystem  TreatAsAtomicUnit=on
  Idle-Loop State Machine Tilt : Stateflow chart  TreatAsAtomicUnit=on
  wires:
  Function-Call Generator/1 -> Function-Call Subsystem/Trigger

== system Target_Control_System/Target_Control_System/MainLoop/tiltMotor_mainLoop/Decimation gate for 200 Hz Tilt ==
  Function-Call Generator : simulink/Ports & Subsystems/Function-Call Generator  sample_time=-1  numberOfIterations=1  DisallowWideOutput=off
  motorTaskMainDecimationAStep(&oTilt) : Subsystem  TreatAsAtomicUnit=on
  wires:
  Function-Call Generator/1 -> motorTaskMainDecimationAStep(&oTilt)/Trigger

== system Target_Control_System/Target_Control_System/MainLoop/tiltMotor_mainLoop/Decimation gate for 5000 Hz Tilt ==
  Function-Call Generator : simulink/Ports & Subsystems/Function-Call Generator  sample_time=-1  numberOfIterations=1  DisallowWideOutput=off
  motorTaskProcessExternalSetpoints(&oTilt) : Subsystem  TreatAsAtomicUnit=on
  wires:
  Function-Call Generator/1 -> motorTaskProcessExternalSetpoints(&oTilt)/Trigger

== system Target_Control_System/Target_Control_System/MainLoop/tiltMotor_mainLoop/mainTask_tilt ==
  Constant8 : Constant  Value=TARGET_CODE_GEN  SampleTime=-1
  Function-Call Split1 : FunctionCallSplit  NumOutputPorts=2
  Function-Call Split10 : FunctionCallSplit  NumOutputPorts=2
  NOT : Logic  Operator=NOT  IconShape=distinctive  AllPortsSameDT=off  OutDataTypeStr=boolean
  PWM for Simulation : Subsystem  TreatAsAtomicUnit=on
  Variant Subsystem : Subsystem  Variant=on
  motorTaskMainFastStep(&oTilt) : Subsystem  TreatAsAtomicUnit=on
  motorTaskManagePwmRequestFlags(&oTilt) : Subsystem
  resetFlag_uiDataFromIsrToMainUpdated : Subsystem
  Out1 : Outport
  wires:
  Constant8/1 -> NOT/1
  NOT/1 -> PWM for Simulation/Enable
  PWM for Simulation/1(Out1) -> Out1/1  "tiltMotor_PWMticks"
  Function-Call Split10/1 -> motorTaskMainFastStep(&oTilt)/Trigger
  Function-Call Split1/2 -> resetFlag_uiDataFromIsrToMainUpdated/Trigger
  Function-Call Split1/1 -> motorTaskManagePwmRequestFlags(&oTilt)/Trigger
  Function-Call Split10/2 -> Function-Call Split1/1
  Variant Subsystem/1(Out1) -> Function-Call Split10/1

== system Target_Control_System/Target_Control_System/ModelSource/IncludeCustomCode/Model Source ==

== system Target_Control_System/Target_Control_System/Simulation Controls/Simulation Data Store Initialization/initializationFlowControl ==
  Trigger : TriggerPort  TriggerType=falling  VariantControl=(inherit)
  Constant : Constant  Commented=on  Value=0  OutDataTypeStr=uint32  SampleTime=-1
  Data Store Write : DataStoreWrite  Commented=on  DataStoreName=fpga_uiPWMInterruptCount_  IndexOptions=Index vector (dialog)  Indices=1  OutputSizes=1
  Data Store Write6 : DataStoreWrite  Commented=on  DataStoreName=mdl_suiIsrSmallInvCounter_  IndexOptions=Index vector (dialog)  Indices=1  OutputSizes=1
  Function-Call Generator : simulink/Ports & Subsystems/Function-Call Generator  sample_time=-1  numberOfIterations=1  DisallowWideOutput=off
  Out1 : Outport
  wires:
  Constant/1 -> Data Store Write6/1, Data Store Write/1
  Function-Call Generator/1 -> Out1/1

== system Target_Control_System/Target_Control_System/Simulation Controls/Simulation Data Store Initialization/initializeDataForPitch() ==
  initializeDataForPitch : TriggerPort  TriggerType=function-call  VariantControl=(inherit)  OutputDataType=int8
  initializeHardwareInvPitch() : Subsystem
  initializeIntTaskParametersPitch() : Subsystem
  initializeMotorTaskParameterPitch() : Subsystem

== system Target_Control_System/Target_Control_System/Simulation Controls/Simulation Data Store Initialization/initializeDataForTilt() ==
  initializeDataForTilt : TriggerPort  TriggerType=function-call  VariantControl=(inherit)  OutputDataType=int8
  Function-Call Generator : simulink/Ports & Subsystems/Function-Call Generator  sample_time=-1  numberOfIterations=1  DisallowWideOutput=off
  Function-Call Split1 : FunctionCallSplit  NumOutputPorts=2
  Function-Call Split10 : FunctionCallSplit  NumOutputPorts=2
  initializeHardwareInvTilt : Subsystem  TreatAsAtomicUnit=on
  initializeIntTaskParametersTilt : Subsystem  TreatAsAtomicUnit=on
  initializeMotorTaskParametersTilt : Subsystem  TreatAsAtomicUnit=on
  wires:
  Function-Call Split1/2 -> initializeHardwareInvTilt/Trigger
  Function-Call Split10/2 -> Function-Call Split1/1
  Function-Call Split1/1 -> initializeMotorTaskParametersTilt/Trigger
  Function-Call Generator/1 -> Function-Call Split10/1
  Function-Call Split10/1 -> initializeIntTaskParametersTilt/Trigger

== system Target_Control_System/Target_Control_System/Simulation Controls/Simulation Data Store Initialization/initializeTiltAsMaster() ==
  initializeTiltAsMaster() : TriggerPort  TriggerType=function-call  VariantControl=(inherit)  OutputDataType=int8
  Constant : Constant  Value=0  OutDataTypeStr=uint32  SampleTime=-1
  Data Store Write : DataStoreWrite  DataStoreName=oTilt  DataStoreElements=oTilt.oMot_.oParam_.uiSlaveRole_  IndexOptions=Index vector (dialog)  Indices=1  OutputSizes=1
  wires:
  Constant/1 -> Data Store Write/1

== system Target_Control_System/Target_Control_System/Simulation Controls/Simulation Data Store Initialization/parameter_init_prop ==
  initializeDataForPropulsion : TriggerPort  TriggerType=function-call  VariantControl=(inherit)  OutputDataType=int8
  initializeHardwareInvPropulsion() : Subsystem
  initializeIntTaskParametersPropulsion() : Subsystem
  initializeMotorTaskParameterPropulsion() : Subsystem

== system Target_Control_System/Target_Control_System/Simulation Controls/Simulation Data Store Initialization/parameter_init_pump ==
  initializeDataForPump : TriggerPort  TriggerType=function-call  VariantControl=(inherit)  OutputDataType=int8
  initializeHardwareInvPump() : Subsystem
  initializeIntTaskParametersPump() : Subsystem
  initializeMotorTaskParameterPump() : Subsystem

== system Target_Control_System/Target_Control_System/Simulation Controls/Simulation Data Store Initialization/setHardwareCurrentLimitTilt()1 ==
  setHardwareCurrentLimitTilt : TriggerPort  TriggerType=function-call  VariantControl=Variant

== system Target_Control_System/Target_Control_System/Simulation Controls/Simulation Data Store Initialization/setPositionControlModeTilt() ==
  setPositionControlModeTilt : TriggerPort  TriggerType=function-call  VariantControl=(inherit)  OutputDataType=int8
  Data Store Read : DataStoreRead  DataStoreName=oTilt  DataStoreElements=oTilt.oMot_.oParam_.ePositionControlMode_  IndexOptions=Index vector (dialog)  Indices=1  OutputSizes=1
  Enabled Subsystem : Subsystem  TreatAsAtomicUnit=on
  Enumerated Constant : simulink/Sources/Enumerated Constant  OutDataTypeStr=Enum: EPositionControlModes_t  Value=EPositionControlModes_t.ePassiveHolding  SampleTime=-1
  Equal : RelationalOperator  Operator===  OutDataTypeStr=boolean  RndMeth=Simplest
  NOT : Logic  Operator=NOT  AllPortsSameDT=off  OutDataTypeStr=boolean
  wires:
  Data Store Read/1 -> Equal/1
  Equal/1 -> NOT/1
  NOT/1 -> Enabled Subsystem/Enable
  Enumerated Constant/1 -> Equal/2

== system Target_Control_System/Target_Control_System/Simulation Controls/Simulation Data Store Initialization/setTiltMotorSpecificParameters() ==
  setTiltMotorSpecificParameters() : TriggerPort  TriggerType=function-call  VariantControl=(inherit)  OutputDataType=int8
  Data Store Read : DataStoreRead  DataStoreName=oTilt  DataStoreElements=oTilt.oMot_.oParam_.eInverterAssignment_  IndexOptions=Index vector (dialog)  Indices=1  OutputSizes=1
  Enabled Subsystem MotorType : Subsystem  TreatAsAtomicUnit=on
  Enumerated Constant : simulink/Sources/Enumerated Constant  OutDataTypeStr=Enum: EInverterNames_t  Value=EInverterNames_t.eTilt  SampleTime=-1
  Equal : RelationalOperator  Operator===  OutDataTypeStr=boolean  RndMeth=Simplest
  wires:
  Data Store Read/1 -> Equal/1
  Equal/1 -> Enabled Subsystem MotorType/Enable
  Enumerated Constant/1 -> Equal/2
